simulink model "MotorController"  (R2022a)
settings: Solver=VariableStepAuto  StartTime=0.0  StopTime=10.0  RelTol=1e-3
settings Model: Creator=Lenovo  LastModifiedBy=Lenovo

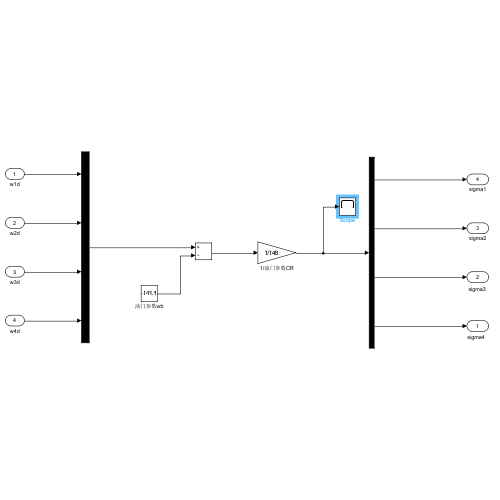
[thumbnail: Simulink's stored preview of the top-level diagram]
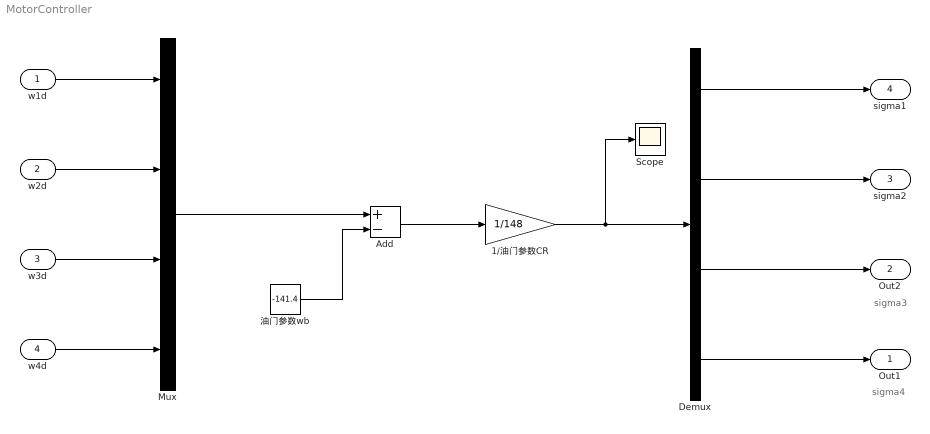
== system MotorController ==
  note: sigma4
  note: sigma3
  w1d : Inport
  w2d : Inport  Port=2
  w3d : Inport  Port=3
  w4d : Inport  Port=4
  1/油门参数CR : Gain  Gain=1/148
  Add : Sum  Inputs=+-
  Demux : Demux
  Mux : Mux
  Scope : Scope
  油门参数wb : Constant  Value=-141.4
  Out1 : Outport
  Out2 : Outport  Port=2
  sigma2 : Outport  Port=3
  sigma1 : Outport  Port=4
  wires:
  w3d/1 -> Mux/3
  w4d/1 -> Mux/4
  w2d/1 -> Mux/2
  w1d/1 -> Mux/1
  油门参数wb/1 -> Add/2
  Mux/1 -> Add/1
  Add/1 -> 1/油门参数CR/1
  1/油门参数CR/1 -> Scope/1, Demux/1
  Demux/4 -> Out1/1
  Demux/3 -> Out2/1
  Demux/2 -> sigma2/1
  Demux/1 -> sigma1/1
